simulink model "simulator_prototype_v3_pdg"  (R2021b)
settings: Solver=VariableStepAuto  StartTime=0.0  StopTime=60  FixedStep=0.0001  RelTol=1e-4
undefined symbols (not defined in the file or in its folder): X, Y, Z
libraries: sm_lib x47, nesl_utility x7, simulink x1
(part 13 of 13)

== matlab function simulator_prototype_v3_pdg/Energy Analysis/MATLAB Function ==
  data: dq input; T output; H input
function T = Kinetic_Energy(dq, H)
T = real((1/2)*transpose(dq)*H*dq);
